simulink model "canTransceiverModel"  (R2018a)
settings: Solver=FixedStepDiscrete  StartTime=0.0  StopTime=50  RelTol=1e-3  EnableMultiTasking=on
values from neighbouring files (symbols this model uses):
  sampleTime = 0.040    (= 0.04)    [canTrasceiverConfig.m]
  sensorLocationConfig = uint8(sensorLocationConfig)    [canTrasceiverConfig.m]
undefined symbols (not defined in the file or in its folder): canChannel, CRC
libraries: simulink x81, canmsglib x27, canlib x8, commcrc2 x1
(part 5 of 5)

== system canTransceiverModel/BH-CAN Sensor 3 Output/Targets 0-9 (ID 0x300-309)/Targets Range and Bearing Information/Information Target 7/Target Format 2/Sensor number/Mod 16 ==
  Input : Inport
  Constant : Constant  Value=16  OutDataTypeStr=Inherit: Inherit via back propagation
  Rem : Math  Operator=mod  OutputSignalType=real  SaturateOnIntegerOverflow=on
  Output : Outport
  wires:
  Input/1 -> Rem/1
  Constant/1 -> Rem/2
  Rem/1 -> Output/1

== system canTransceiverModel/BH-CAN Sensor 3 Output/Targets 0-9 (ID 0x300-309)/Targets Range and Bearing Information/Information Target 8/Target Format 2/Bearing/Divide by 5 ==
  Dividend : Inport
  Constant1 : Constant  Value=5  OutDataTypeStr=Inherit: Inherit via back propagation
  Divide : Product  Inputs=*/  OutDataTypeStr=single
  Result : Outport
  wires:
  Constant1/1 -> Divide/2
  Divide/1 -> Result/1
  Dividend/1 -> Divide/1

== system canTransceiverModel/BH-CAN Sensor 3 Output/Targets 0-9 (ID 0x300-309)/Targets Range and Bearing Information/Information Target 8/Target Format 2/Bearing/Mod 4 ==
  Input : Inport
  Constant : Constant  Value=4  OutDataTypeStr=Inherit: Inherit via back propagation
  Rem : Math  Operator=mod  OutputSignalType=real  SaturateOnIntegerOverflow=on
  Output : Outport
  wires:
  Input/1 -> Rem/1
  Constant/1 -> Rem/2
  Rem/1 -> Output/1

== system canTransceiverModel/BH-CAN Sensor 3 Output/Targets 0-9 (ID 0x300-309)/Targets Range and Bearing Information/Information Target 8/Target Format 2/Range/Divide by 100 ==
  Dividend : Inport
  Constant1 : Constant  Value=100  OutDataTypeStr=Inherit: Inherit via back propagation
  Divide : Product  Inputs=*/  OutDataTypeStr=single
  Result : Outport
  wires:
  Constant1/1 -> Divide/2
  Divide/1 -> Result/1
  Dividend/1 -> Divide/1

== system canTransceiverModel/BH-CAN Sensor 3 Output/Targets 0-9 (ID 0x300-309)/Targets Range and Bearing Information/Information Target 8/Target Format 2/Range/Divide by 16 ==
  Dividend : Inport
  Constant1 : Constant  Value=16  OutDataTypeStr=Inherit: Inherit via back propagation
  Divide : Product  Inputs=*/
  Result : Outport
  wires:
  Constant1/1 -> Divide/2
  Dividend/1 -> Divide/1
  Divide/1 -> Result/1

== system canTransceiverModel/BH-CAN Sensor 3 Output/Targets 0-9 (ID 0x300-309)/Targets Range and Bearing Information/Information Target 8/Target Format 2/Sensor number/Mod 16 ==
  Input : Inport
  Constant : Constant  Value=16  OutDataTypeStr=Inherit: Inherit via back propagation
  Rem : Math  Operator=mod  OutputSignalType=real  SaturateOnIntegerOverflow=on
  Output : Outport
  wires:
  Input/1 -> Rem/1
  Constant/1 -> Rem/2
  Rem/1 -> Output/1

== system canTransceiverModel/BH-CAN Sensor 3 Output/Targets 0-9 (ID 0x300-309)/Targets Range and Bearing Information/Information Target 9/Target Format 2/Bearing/Divide by 5 ==
  Dividend : Inport
  Constant1 : Constant  Value=5  OutDataTypeStr=Inherit: Inherit via back propagation
  Divide : Product  Inputs=*/  OutDataTypeStr=single
  Result : Outport
  wires:
  Constant1/1 -> Divide/2
  Divide/1 -> Result/1
  Dividend/1 -> Divide/1

== system canTransceiverModel/BH-CAN Sensor 3 Output/Targets 0-9 (ID 0x300-309)/Targets Range and Bearing Information/Information Target 9/Target Format 2/Bearing/Mod 4 ==
  Input : Inport
  Constant : Constant  Value=4  OutDataTypeStr=Inherit: Inherit via back propagation
  Rem : Math  Operator=mod  OutputSignalType=real  SaturateOnIntegerOverflow=on
  Output : Outport
  wires:
  Input/1 -> Rem/1
  Constant/1 -> Rem/2
  Rem/1 -> Output/1

== system canTransceiverModel/BH-CAN Sensor 3 Output/Targets 0-9 (ID 0x300-309)/Targets Range and Bearing Information/Information Target 9/Target Format 2/Range/Divide by 100 ==
  Dividend : Inport
  Constant1 : Constant  Value=100  OutDataTypeStr=Inherit: Inherit via back propagation
  Divide : Product  Inputs=*/  OutDataTypeStr=single
  Result : Outport
  wires:
  Constant1/1 -> Divide/2
  Divide/1 -> Result/1
  Dividend/1 -> Divide/1

== system canTransceiverModel/BH-CAN Sensor 3 Output/Targets 0-9 (ID 0x300-309)/Targets Range and Bearing Information/Information Target 9/Target Format 2/Range/Divide by 16 ==
  Dividend : Inport
  Constant1 : Constant  Value=16  OutDataTypeStr=Inherit: Inherit via back propagation
  Divide : Product  Inputs=*/
  Result : Outport
  wires:
  Constant1/1 -> Divide/2
  Dividend/1 -> Divide/1
  Divide/1 -> Result/1

== system canTransceiverModel/BH-CAN Sensor 3 Output/Targets 0-9 (ID 0x300-309)/Targets Range and Bearing Information/Information Target 9/Target Format 2/Sensor number/Mod 16 ==
  Input : Inport
  Constant : Constant  Value=16  OutDataTypeStr=Inherit: Inherit via back propagation
  Rem : Math  Operator=mod  OutputSignalType=real  SaturateOnIntegerOverflow=on
  Output : Outport
  wires:
  Input/1 -> Rem/1
  Constant/1 -> Rem/2
  Rem/1 -> Output/1

== system canTransceiverModel/BH-CAN Sensor 4 Output/Targets 0-9 (ID 0x300-309)/Targets Range and Bearing Information/Information Target 0/Target Format 2/Bearing/Divide by 5 ==
  Dividend : Inport
  Constant1 : Constant  Value=5  OutDataTypeStr=Inherit: Inherit via back propagation
  Divide : Product  Inputs=*/  OutDataTypeStr=single
  Result : Outport
  wires:
  Constant1/1 -> Divide/2
  Divide/1 -> Result/1
  Dividend/1 -> Divide/1

== system canTransceiverModel/BH-CAN Sensor 4 Output/Targets 0-9 (ID 0x300-309)/Targets Range and Bearing Information/Information Target 0/Target Format 2/Bearing/Mod 4 ==
  Input : Inport
  Constant : Constant  Value=4  OutDataTypeStr=Inherit: Inherit via back propagation
  Rem : Math  Operator=mod  OutputSignalType=real  SaturateOnIntegerOverflow=on
  Output : Outport
  wires:
  Input/1 -> Rem/1
  Constant/1 -> Rem/2
  Rem/1 -> Output/1

== system canTransceiverModel/BH-CAN Sensor 4 Output/Targets 0-9 (ID 0x300-309)/Targets Range and Bearing Information/Information Target 0/Target Format 2/Range/Divide by 100 ==
  Dividend : Inport
  Constant1 : Constant  Value=100  OutDataTypeStr=Inherit: Inherit via back propagation
  Divide : Product  Inputs=*/  OutDataTypeStr=single
  Result : Outport
  wires:
  Constant1/1 -> Divide/2
  Divide/1 -> Result/1
  Dividend/1 -> Divide/1

== system canTransceiverModel/BH-CAN Sensor 4 Output/Targets 0-9 (ID 0x300-309)/Targets Range and Bearing Information/Information Target 0/Target Format 2/Range/Divide by 16 ==
  Dividend : Inport
  Constant1 : Constant  Value=16  OutDataTypeStr=Inherit: Inherit via back propagation
  Divide : Product  Inputs=*/
  Result : Outport
  wires:
  Constant1/1 -> Divide/2
  Dividend/1 -> Divide/1
  Divide/1 -> Result/1

== system canTransceiverModel/BH-CAN Sensor 4 Output/Targets 0-9 (ID 0x300-309)/Targets Range and Bearing Information/Information Target 0/Target Format 2/Sensor number/Mod 16 ==
  Input : Inport
  Constant : Constant  Value=16  OutDataTypeStr=Inherit: Inherit via back propagation
  Rem : Math  Operator=mod  OutputSignalType=real  SaturateOnIntegerOverflow=on
  Output : Outport
  wires:
  Input/1 -> Rem/1
  Constant/1 -> Rem/2
  Rem/1 -> Output/1

== system canTransceiverModel/BH-CAN Sensor 4 Output/Targets 0-9 (ID 0x300-309)/Targets Range and Bearing Information/Information Target 1/Target Format 2/Bearing/Divide by 5 ==
  Dividend : Inport
  Constant1 : Constant  Value=5  OutDataTypeStr=Inherit: Inherit via back propagation
  Divide : Product  Inputs=*/  OutDataTypeStr=single
  Result : Outport
  wires:
  Constant1/1 -> Divide/2
  Divide/1 -> Result/1
  Dividend/1 -> Divide/1

== system canTransceiverModel/BH-CAN Sensor 4 Output/Targets 0-9 (ID 0x300-309)/Targets Range and Bearing Information/Information Target 1/Target Format 2/Bearing/Mod 4 ==
  Input : Inport
  Constant : Constant  Value=4  OutDataTypeStr=Inherit: Inherit via back propagation
  Rem : Math  Operator=mod  OutputSignalType=real  SaturateOnIntegerOverflow=on
  Output : Outport
  wires:
  Input/1 -> Rem/1
  Constant/1 -> Rem/2
  Rem/1 -> Output/1

== system canTransceiverModel/BH-CAN Sensor 4 Output/Targets 0-9 (ID 0x300-309)/Targets Range and Bearing Information/Information Target 1/Target Format 2/Range/Divide by 100 ==
  Dividend : Inport
  Constant1 : Constant  Value=100  OutDataTypeStr=Inherit: Inherit via back propagation
  Divide : Product  Inputs=*/  OutDataTypeStr=single
  Result : Outport
  wires:
  Constant1/1 -> Divide/2
  Divide/1 -> Result/1
  Dividend/1 -> Divide/1

== system canTransceiverModel/BH-CAN Sensor 4 Output/Targets 0-9 (ID 0x300-309)/Targets Range and Bearing Information/Information Target 1/Target Format 2/Range/Divide by 16 ==
  Dividend : Inport
  Constant1 : Constant  Value=16  OutDataTypeStr=Inherit: Inherit via back propagation
  Divide : Product  Inputs=*/
  Result : Outport
  wires:
  Constant1/1 -> Divide/2
  Dividend/1 -> Divide/1
  Divide/1 -> Result/1

== system canTransceiverModel/BH-CAN Sensor 4 Output/Targets 0-9 (ID 0x300-309)/Targets Range and Bearing Information/Information Target 1/Target Format 2/Sensor number/Mod 16 ==
  Input : Inport
  Constant : Constant  Value=16  OutDataTypeStr=Inherit: Inherit via back propagation
  Rem : Math  Operator=mod  OutputSignalType=real  SaturateOnIntegerOverflow=on
  Output : Outport
  wires:
  Input/1 -> Rem/1
  Constant/1 -> Rem/2
  Rem/1 -> Output/1

== system canTransceiverModel/BH-CAN Sensor 4 Output/Targets 0-9 (ID 0x300-309)/Targets Range and Bearing Information/Information Target 2/Target Format 2/Bearing/Divide by 5 ==
  Dividend : Inport
  Constant1 : Constant  Value=5  OutDataTypeStr=Inherit: Inherit via back propagation
  Divide : Product  Inputs=*/  OutDataTypeStr=single
  Result : Outport
  wires:
  Constant1/1 -> Divide/2
  Divide/1 -> Result/1
  Dividend/1 -> Divide/1

== system canTransceiverModel/BH-CAN Sensor 4 Output/Targets 0-9 (ID 0x300-309)/Targets Range and Bearing Information/Information Target 2/Target Format 2/Bearing/Mod 4 ==
  Input : Inport
  Constant : Constant  Value=4  OutDataTypeStr=Inherit: Inherit via back propagation
  Rem : Math  Operator=mod  OutputSignalType=real  SaturateOnIntegerOverflow=on
  Output : Outport
  wires:
  Input/1 -> Rem/1
  Constant/1 -> Rem/2
  Rem/1 -> Output/1

== system canTransceiverModel/BH-CAN Sensor 4 Output/Targets 0-9 (ID 0x300-309)/Targets Range and Bearing Information/Information Target 2/Target Format 2/Range/Divide by 100 ==
  Dividend : Inport
  Constant1 : Constant  Value=100  OutDataTypeStr=Inherit: Inherit via back propagation
  Divide : Product  Inputs=*/  OutDataTypeStr=single
  Result : Outport
  wires:
  Constant1/1 -> Divide/2
  Divide/1 -> Result/1
  Dividend/1 -> Divide/1

== system canTransceiverModel/BH-CAN Sensor 4 Output/Targets 0-9 (ID 0x300-309)/Targets Range and Bearing Information/Information Target 2/Target Format 2/Range/Divide by 16 ==
  Dividend : Inport
  Constant1 : Constant  Value=16  OutDataTypeStr=Inherit: Inherit via back propagation
  Divide : Product  Inputs=*/
  Result : Outport
  wires:
  Constant1/1 -> Divide/2
  Dividend/1 -> Divide/1
  Divide/1 -> Result/1

== system canTransceiverModel/BH-CAN Sensor 4 Output/Targets 0-9 (ID 0x300-309)/Targets Range and Bearing Information/Information Target 2/Target Format 2/Sensor number/Mod 16 ==
  Input : Inport
  Constant : Constant  Value=16  OutDataTypeStr=Inherit: Inherit via back propagation
  Rem : Math  Operator=mod  OutputSignalType=real  SaturateOnIntegerOverflow=on
  Output : Outport
  wires:
  Input/1 -> Rem/1
  Constant/1 -> Rem/2
  Rem/1 -> Output/1

== system canTransceiverModel/BH-CAN Sensor 4 Output/Targets 0-9 (ID 0x300-309)/Targets Range and Bearing Information/Information Target 3/Target Format 2/Bearing/Divide by 5 ==
  Dividend : Inport
  Constant1 : Constant  Value=5  OutDataTypeStr=Inherit: Inherit via back propagation
  Divide : Product  Inputs=*/  OutDataTypeStr=single
  Result : Outport
  wires:
  Constant1/1 -> Divide/2
  Divide/1 -> Result/1
  Dividend/1 -> Divide/1

== system canTransceiverModel/BH-CAN Sensor 4 Output/Targets 0-9 (ID 0x300-309)/Targets Range and Bearing Information/Information Target 3/Target Format 2/Bearing/Mod 4 ==
  Input : Inport
  Constant : Constant  Value=4  OutDataTypeStr=Inherit: Inherit via back propagation
  Rem : Math  Operator=mod  OutputSignalType=real  SaturateOnIntegerOverflow=on
  Output : Outport
  wires:
  Input/1 -> Rem/1
  Constant/1 -> Rem/2
  Rem/1 -> Output/1

== system canTransceiverModel/BH-CAN Sensor 4 Output/Targets 0-9 (ID 0x300-309)/Targets Range and Bearing Information/Information Target 3/Target Format 2/Range/Divide by 100 ==
  Dividend : Inport
  Constant1 : Constant  Value=100  OutDataTypeStr=Inherit: Inherit via back propagation
  Divide : Product  Inputs=*/  OutDataTypeStr=single
  Result : Outport
  wires:
  Constant1/1 -> Divide/2
  Divide/1 -> Result/1
  Dividend/1 -> Divide/1

== system canTransceiverModel/BH-CAN Sensor 4 Output/Targets 0-9 (ID 0x300-309)/Targets Range and Bearing Information/Information Target 3/Target Format 2/Range/Divide by 16 ==
  Dividend : Inport
  Constant1 : Constant  Value=16  OutDataTypeStr=Inherit: Inherit via back propagation
  Divide : Product  Inputs=*/
  Result : Outport
  wires:
  Constant1/1 -> Divide/2
  Dividend/1 -> Divide/1
  Divide/1 -> Result/1

== system canTransceiverModel/BH-CAN Sensor 4 Output/Targets 0-9 (ID 0x300-309)/Targets Range and Bearing Information/Information Target 3/Target Format 2/Sensor number/Mod 16 ==
  Input : Inport
  Constant : Constant  Value=16  OutDataTypeStr=Inherit: Inherit via back propagation
  Rem : Math  Operator=mod  OutputSignalType=real  SaturateOnIntegerOverflow=on
  Output : Outport
  wires:
  Input/1 -> Rem/1
  Constant/1 -> Rem/2
  Rem/1 -> Output/1

== system canTransceiverModel/BH-CAN Sensor 4 Output/Targets 0-9 (ID 0x300-309)/Targets Range and Bearing Information/Information Target 4/Target Format 2/Bearing/Divide by 5 ==
  Dividend : Inport
  Constant1 : Constant  Value=5  OutDataTypeStr=Inherit: Inherit via back propagation
  Divide : Product  Inputs=*/  OutDataTypeStr=single
  Result : Outport
  wires:
  Constant1/1 -> Divide/2
  Divide/1 -> Result/1
  Dividend/1 -> Divide/1

== system canTransceiverModel/BH-CAN Sensor 4 Output/Targets 0-9 (ID 0x300-309)/Targets Range and Bearing Information/Information Target 4/Target Format 2/Bearing/Mod 4 ==
  Input : Inport
  Constant : Constant  Value=4  OutDataTypeStr=Inherit: Inherit via back propagation
  Rem : Math  Operator=mod  OutputSignalType=real  SaturateOnIntegerOverflow=on
  Output : Outport
  wires:
  Input/1 -> Rem/1
  Constant/1 -> Rem/2
  Rem/1 -> Output/1

== system canTransceiverModel/BH-CAN Sensor 4 Output/Targets 0-9 (ID 0x300-309)/Targets Range and Bearing Information/Information Target 4/Target Format 2/Range/Divide by 100 ==
  Dividend : Inport
  Constant1 : Constant  Value=100  OutDataTypeStr=Inherit: Inherit via back propagation
  Divide : Product  Inputs=*/  OutDataTypeStr=single
  Result : Outport
  wires:
  Constant1/1 -> Divide/2
  Divide/1 -> Result/1
  Dividend/1 -> Divide/1

== system canTransceiverModel/BH-CAN Sensor 4 Output/Targets 0-9 (ID 0x300-309)/Targets Range and Bearing Information/Information Target 4/Target Format 2/Range/Divide by 16 ==
  Dividend : Inport
  Constant1 : Constant  Value=16  OutDataTypeStr=Inherit: Inherit via back propagation
  Divide : Product  Inputs=*/
  Result : Outport
  wires:
  Constant1/1 -> Divide/2
  Dividend/1 -> Divide/1
  Divide/1 -> Result/1

== system canTransceiverModel/BH-CAN Sensor 4 Output/Targets 0-9 (ID 0x300-309)/Targets Range and Bearing Information/Information Target 4/Target Format 2/Sensor number/Mod 16 ==
  Input : Inport
  Constant : Constant  Value=16  OutDataTypeStr=Inherit: Inherit via back propagation
  Rem : Math  Operator=mod  OutputSignalType=real  SaturateOnIntegerOverflow=on
  Output : Outport
  wires:
  Input/1 -> Rem/1
  Constant/1 -> Rem/2
  Rem/1 -> Output/1

== system canTransceiverModel/BH-CAN Sensor 4 Output/Targets 0-9 (ID 0x300-309)/Targets Range and Bearing Information/Information Target 5/Target Format 2/Bearing/Divide by 5 ==
  Dividend : Inport
  Constant1 : Constant  Value=5  OutDataTypeStr=Inherit: Inherit via back propagation
  Divide : Product  Inputs=*/  OutDataTypeStr=single
  Result : Outport
  wires:
  Constant1/1 -> Divide/2
  Divide/1 -> Result/1
  Dividend/1 -> Divide/1

== system canTransceiverModel/BH-CAN Sensor 4 Output/Targets 0-9 (ID 0x300-309)/Targets Range and Bearing Information/Information Target 5/Target Format 2/Bearing/Mod 4 ==
  Input : Inport
  Constant : Constant  Value=4  OutDataTypeStr=Inherit: Inherit via back propagation
  Rem : Math  Operator=mod  OutputSignalType=real  SaturateOnIntegerOverflow=on
  Output : Outport
  wires:
  Input/1 -> Rem/1
  Constant/1 -> Rem/2
  Rem/1 -> Output/1

== system canTransceiverModel/BH-CAN Sensor 4 Output/Targets 0-9 (ID 0x300-309)/Targets Range and Bearing Information/Information Target 5/Target Format 2/Range/Divide by 100 ==
  Dividend : Inport
  Constant1 : Constant  Value=100  OutDataTypeStr=Inherit: Inherit via back propagation
  Divide : Product  Inputs=*/  OutDataTypeStr=single
  Result : Outport
  wires:
  Constant1/1 -> Divide/2
  Divide/1 -> Result/1
  Dividend/1 -> Divide/1

== system canTransceiverModel/BH-CAN Sensor 4 Output/Targets 0-9 (ID 0x300-309)/Targets Range and Bearing Information/Information Target 5/Target Format 2/Range/Divide by 16 ==
  Dividend : Inport
  Constant1 : Constant  Value=16  OutDataTypeStr=Inherit: Inherit via back propagation
  Divide : Product  Inputs=*/
  Result : Outport
  wires:
  Constant1/1 -> Divide/2
  Dividend/1 -> Divide/1
  Divide/1 -> Result/1

== system canTransceiverModel/BH-CAN Sensor 4 Output/Targets 0-9 (ID 0x300-309)/Targets Range and Bearing Information/Information Target 5/Target Format 2/Sensor number/Mod 16 ==
  Input : Inport
  Constant : Constant  Value=16  OutDataTypeStr=Inherit: Inherit via back propagation
  Rem : Math  Operator=mod  OutputSignalType=real  SaturateOnIntegerOverflow=on
  Output : Outport
  wires:
  Input/1 -> Rem/1
  Constant/1 -> Rem/2
  Rem/1 -> Output/1

== system canTransceiverModel/BH-CAN Sensor 4 Output/Targets 0-9 (ID 0x300-309)/Targets Range and Bearing Information/Information Target 6/Target Format 2/Bearing/Divide by 5 ==
  Dividend : Inport
  Constant1 : Constant  Value=5  OutDataTypeStr=Inherit: Inherit via back propagation
  Divide : Product  Inputs=*/  OutDataTypeStr=single
  Result : Outport
  wires:
  Constant1/1 -> Divide/2
  Divide/1 -> Result/1
  Dividend/1 -> Divide/1

== system canTransceiverModel/BH-CAN Sensor 4 Output/Targets 0-9 (ID 0x300-309)/Targets Range and Bearing Information/Information Target 6/Target Format 2/Bearing/Mod 4 ==
  Input : Inport
  Constant : Constant  Value=4  OutDataTypeStr=Inherit: Inherit via back propagation
  Rem : Math  Operator=mod  OutputSignalType=real  SaturateOnIntegerOverflow=on
  Output : Outport
  wires:
  Input/1 -> Rem/1
  Constant/1 -> Rem/2
  Rem/1 -> Output/1

== system canTransceiverModel/BH-CAN Sensor 4 Output/Targets 0-9 (ID 0x300-309)/Targets Range and Bearing Information/Information Target 6/Target Format 2/Range/Divide by 100 ==
  Dividend : Inport
  Constant1 : Constant  Value=100  OutDataTypeStr=Inherit: Inherit via back propagation
  Divide : Product  Inputs=*/  OutDataTypeStr=single
  Result : Outport
  wires:
  Constant1/1 -> Divide/2
  Divide/1 -> Result/1
  Dividend/1 -> Divide/1

== system canTransceiverModel/BH-CAN Sensor 4 Output/Targets 0-9 (ID 0x300-309)/Targets Range and Bearing Information/Information Target 6/Target Format 2/Range/Divide by 16 ==
  Dividend : Inport
  Constant1 : Constant  Value=16  OutDataTypeStr=Inherit: Inherit via back propagation
  Divide : Product  Inputs=*/
  Result : Outport
  wires:
  Constant1/1 -> Divide/2
  Dividend/1 -> Divide/1
  Divide/1 -> Result/1

== system canTransceiverModel/BH-CAN Sensor 4 Output/Targets 0-9 (ID 0x300-309)/Targets Range and Bearing Information/Information Target 6/Target Format 2/Sensor number/Mod 16 ==
  Input : Inport
  Constant : Constant  Value=16  OutDataTypeStr=Inherit: Inherit via back propagation
  Rem : Math  Operator=mod  OutputSignalType=real  SaturateOnIntegerOverflow=on
  Output : Outport
  wires:
  Input/1 -> Rem/1
  Constant/1 -> Rem/2
  Rem/1 -> Output/1

== system canTransceiverModel/BH-CAN Sensor 4 Output/Targets 0-9 (ID 0x300-309)/Targets Range and Bearing Information/Information Target 7/Target Format 2/Bearing/Divide by 5 ==
  Dividend : Inport
  Constant1 : Constant  Value=5  OutDataTypeStr=Inherit: Inherit via back propagation
  Divide : Product  Inputs=*/  OutDataTypeStr=single
  Result : Outport
  wires:
  Constant1/1 -> Divide/2
  Divide/1 -> Result/1
  Dividend/1 -> Divide/1

== system canTransceiverModel/BH-CAN Sensor 4 Output/Targets 0-9 (ID 0x300-309)/Targets Range and Bearing Information/Information Target 7/Target Format 2/Bearing/Mod 4 ==
  Input : Inport
  Constant : Constant  Value=4  OutDataTypeStr=Inherit: Inherit via back propagation
  Rem : Math  Operator=mod  OutputSignalType=real  SaturateOnIntegerOverflow=on
  Output : Outport
  wires:
  Input/1 -> Rem/1
  Constant/1 -> Rem/2
  Rem/1 -> Output/1

== system canTransceiverModel/BH-CAN Sensor 4 Output/Targets 0-9 (ID 0x300-309)/Targets Range and Bearing Information/Information Target 7/Target Format 2/Range/Divide by 100 ==
  Dividend : Inport
  Constant1 : Constant  Value=100  OutDataTypeStr=Inherit: Inherit via back propagation
  Divide : Product  Inputs=*/  OutDataTypeStr=single
  Result : Outport
  wires:
  Constant1/1 -> Divide/2
  Divide/1 -> Result/1
  Dividend/1 -> Divide/1

== system canTransceiverModel/BH-CAN Sensor 4 Output/Targets 0-9 (ID 0x300-309)/Targets Range and Bearing Information/Information Target 7/Target Format 2/Range/Divide by 16 ==
  Dividend : Inport
  Constant1 : Constant  Value=16  OutDataTypeStr=Inherit: Inherit via back propagation
  Divide : Product  Inputs=*/
  Result : Outport
  wires:
  Constant1/1 -> Divide/2
  Dividend/1 -> Divide/1
  Divide/1 -> Result/1

== system canTransceiverModel/BH-CAN Sensor 4 Output/Targets 0-9 (ID 0x300-309)/Targets Range and Bearing Information/Information Target 7/Target Format 2/Sensor number/Mod 16 ==
  Input : Inport
  Constant : Constant  Value=16  OutDataTypeStr=Inherit: Inherit via back propagation
  Rem : Math  Operator=mod  OutputSignalType=real  SaturateOnIntegerOverflow=on
  Output : Outport
  wires:
  Input/1 -> Rem/1
  Constant/1 -> Rem/2
  Rem/1 -> Output/1

== system canTransceiverModel/BH-CAN Sensor 4 Output/Targets 0-9 (ID 0x300-309)/Targets Range and Bearing Information/Information Target 8/Target Format 2/Bearing/Divide by 5 ==
  Dividend : Inport
  Constant1 : Constant  Value=5  OutDataTypeStr=Inherit: Inherit via back propagation
  Divide : Product  Inputs=*/  OutDataTypeStr=single
  Result : Outport
  wires:
  Constant1/1 -> Divide/2
  Divide/1 -> Result/1
  Dividend/1 -> Divide/1

== system canTransceiverModel/BH-CAN Sensor 4 Output/Targets 0-9 (ID 0x300-309)/Targets Range and Bearing Information/Information Target 8/Target Format 2/Bearing/Mod 4 ==
  Input : Inport
  Constant : Constant  Value=4  OutDataTypeStr=Inherit: Inherit via back propagation
  Rem : Math  Operator=mod  OutputSignalType=real  SaturateOnIntegerOverflow=on
  Output : Outport
  wires:
  Input/1 -> Rem/1
  Constant/1 -> Rem/2
  Rem/1 -> Output/1

== system canTransceiverModel/BH-CAN Sensor 4 Output/Targets 0-9 (ID 0x300-309)/Targets Range and Bearing Information/Information Target 8/Target Format 2/Range/Divide by 100 ==
  Dividend : Inport
  Constant1 : Constant  Value=100  OutDataTypeStr=Inherit: Inherit via back propagation
  Divide : Product  Inputs=*/  OutDataTypeStr=single
  Result : Outport
  wires:
  Constant1/1 -> Divide/2
  Divide/1 -> Result/1
  Dividend/1 -> Divide/1

== system canTransceiverModel/BH-CAN Sensor 4 Output/Targets 0-9 (ID 0x300-309)/Targets Range and Bearing Information/Information Target 8/Target Format 2/Range/Divide by 16 ==
  Dividend : Inport
  Constant1 : Constant  Value=16  OutDataTypeStr=Inherit: Inherit via back propagation
  Divide : Product  Inputs=*/
  Result : Outport
  wires:
  Constant1/1 -> Divide/2
  Dividend/1 -> Divide/1
  Divide/1 -> Result/1

== system canTransceiverModel/BH-CAN Sensor 4 Output/Targets 0-9 (ID 0x300-309)/Targets Range and Bearing Information/Information Target 8/Target Format 2/Sensor number/Mod 16 ==
  Input : Inport
  Constant : Constant  Value=16  OutDataTypeStr=Inherit: Inherit via back propagation
  Rem : Math  Operator=mod  OutputSignalType=real  SaturateOnIntegerOverflow=on
  Output : Outport
  wires:
  Input/1 -> Rem/1
  Constant/1 -> Rem/2
  Rem/1 -> Output/1

== system canTransceiverModel/BH-CAN Sensor 4 Output/Targets 0-9 (ID 0x300-309)/Targets Range and Bearing Information/Information Target 9/Target Format 2/Bearing/Divide by 5 ==
  Dividend : Inport
  Constant1 : Constant  Value=5  OutDataTypeStr=Inherit: Inherit via back propagation
  Divide : Product  Inputs=*/  OutDataTypeStr=single
  Result : Outport
  wires:
  Constant1/1 -> Divide/2
  Divide/1 -> Result/1
  Dividend/1 -> Divide/1

== system canTransceiverModel/BH-CAN Sensor 4 Output/Targets 0-9 (ID 0x300-309)/Targets Range and Bearing Information/Information Target 9/Target Format 2/Bearing/Mod 4 ==
  Input : Inport
  Constant : Constant  Value=4  OutDataTypeStr=Inherit: Inherit via back propagation
  Rem : Math  Operator=mod  OutputSignalType=real  SaturateOnIntegerOverflow=on
  Output : Outport
  wires:
  Input/1 -> Rem/1
  Constant/1 -> Rem/2
  Rem/1 -> Output/1

== system canTransceiverModel/BH-CAN Sensor 4 Output/Targets 0-9 (ID 0x300-309)/Targets Range and Bearing Information/Information Target 9/Target Format 2/Range/Divide by 100 ==
  Dividend : Inport
  Constant1 : Constant  Value=100  OutDataTypeStr=Inherit: Inherit via back propagation
  Divide : Product  Inputs=*/  OutDataTypeStr=single
  Result : Outport
  wires:
  Constant1/1 -> Divide/2
  Divide/1 -> Result/1
  Dividend/1 -> Divide/1

== system canTransceiverModel/BH-CAN Sensor 4 Output/Targets 0-9 (ID 0x300-309)/Targets Range and Bearing Information/Information Target 9/Target Format 2/Range/Divide by 16 ==
  Dividend : Inport
  Constant1 : Constant  Value=16  OutDataTypeStr=Inherit: Inherit via back propagation
  Divide : Product  Inputs=*/
  Result : Outport
  wires:
  Constant1/1 -> Divide/2
  Dividend/1 -> Divide/1
  Divide/1 -> Result/1

== system canTransceiverModel/BH-CAN Sensor 4 Output/Targets 0-9 (ID 0x300-309)/Targets Range and Bearing Information/Information Target 9/Target Format 2/Sensor number/Mod 16 ==
  Input : Inport
  Constant : Constant  Value=16  OutDataTypeStr=Inherit: Inherit via back propagation
  Rem : Math  Operator=mod  OutputSignalType=real  SaturateOnIntegerOverflow=on
  Output : Outport
  wires:
  Input/1 -> Rem/1
  Constant/1 -> Rem/2
  Rem/1 -> Output/1

== matlab function canTransceiverModel/BH-CAN Input Command (ID 0x203-204)/BH-CAN Input Command 4 (ID 0x204)/Data Channel 1 (15:0) ==
  data: counter input; sensorLocationConfig input; byte1 output; byte2 output
function [byte1, byte2] = dataChannel1(counter, sensorLocationConfig)

switch counter
    case hex2dec('00')
        byte1 = sensorLocationConfig(4, 1);
        byte2 = sensorLocationConfig(4, 2);
    case hex2dec('10')
        byte1 = sensorLocationConfig(4, 3);
        byte2 = sensorLocationConfig(4, 4);
    case hex2dec('20')
        byte1 = sensorLocationConfig(4, 5);
        byte2 = sensorLocationConfig(4, 6);
    case hex2dec('30')
        byte1 = sensorLocationConfig(4, 7);
        byte2 = sensorLocationConfig(4, 8);
    otherwise
        byte1 = uint8(0);
        byte2 = uint8(0);
    
end

end

== matlab function canTransceiverModel/BH-CAN Input Command (ID 0x203-204)/BH-CAN Input Command 3 (ID 0x203)/Data Channel 1 (15:0) ==
  data: counter input; sensorLocationConfig input; byte1 output; byte2 output
function [byte1, byte2] = dataChannel1(counter, sensorLocationConfig)

switch counter
    case hex2dec('00')
        byte1 = sensorLocationConfig(3, 1);
        byte2 = sensorLocationConfig(3, 2);
    case hex2dec('10')
        byte1 = sensorLocationConfig(3, 3);
        byte2 = sensorLocationConfig(3, 4);
    case hex2dec('20')
        byte1 = sensorLocationConfig(3, 5);
        byte2 = sensorLocationConfig(3, 6);
    case hex2dec('30')
        byte1 = sensorLocationConfig(3, 7);
        byte2 = sensorLocationConfig(3, 8);
    otherwise
        byte1 = uint8(0);
        byte2 = uint8(0);
    
end

end
